simulink model "zeta_effect_on_response"  (R2023b)
settings: Solver=VariableStepAuto  StartTime=0.0  StopTime=10.0  RelTol=1e-3
settings Model: Creator=reemb  LastModifiedBy=reemb

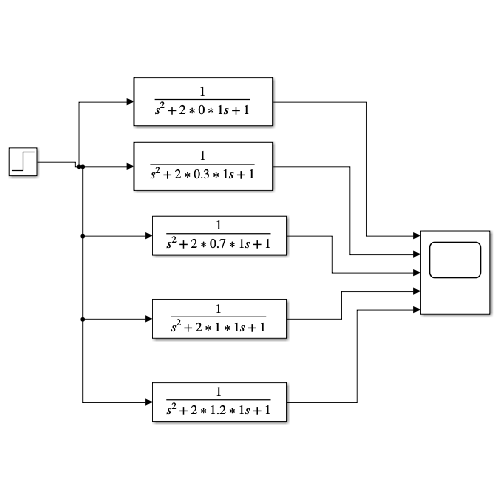
[thumbnail: Simulink's stored preview of the top-level diagram]
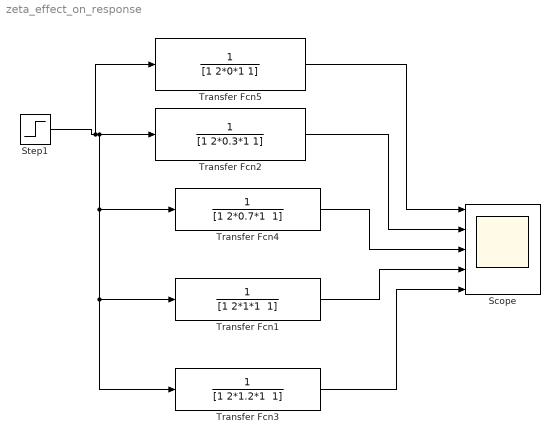
== system zeta_effect_on_response ==
  Scope : Scope  NumInputPorts=5
  Step1 : Step  SampleTime=0
  Transfer Fcn1 : TransferFcn  Denominator="[1 2*1*1  1]"
  Transfer Fcn2 : TransferFcn  Denominator=[1 2*0.3*1 1]
  Transfer Fcn3 : TransferFcn  Denominator="[1 2*1.2*1  1]"
  Transfer Fcn4 : TransferFcn  Denominator="[1 2*0.7*1  1]"
  Transfer Fcn5 : TransferFcn  Denominator=[1 2*0*1 1]
  wires:
  Transfer Fcn4/1 -> Scope/3
  Transfer Fcn2/1 -> Scope/2
  Step1/1 -> Transfer Fcn5/1, Transfer Fcn2/1, Transfer Fcn4/1, Transfer Fcn3/1, Transfer Fcn1/1
  Transfer Fcn1/1 -> Scope/4
  Transfer Fcn3/1 -> Scope/5
  Transfer Fcn5/1 -> Scope/1
